simulink model "Palab3_4_2"  (R2025a)
settings: Solver=ode23t  StartTime=0.0  StopTime=10.0  FixedStep=1  MaxStep=1.1  MinStep=0.9  RelTol=1e-3
settings Model: LastModifiedBy=mieszko
settings SolverCC: InitialStep=1

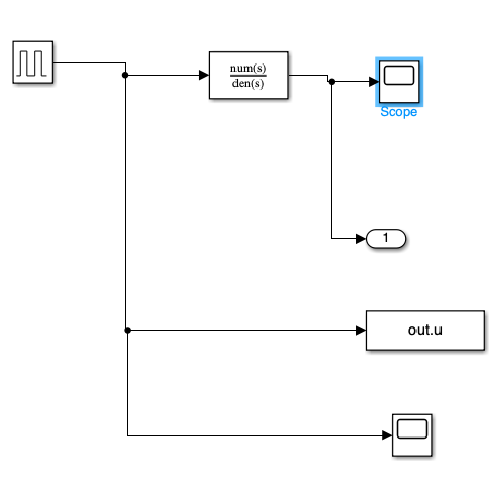
[thumbnail: Simulink's stored preview of the top-level diagram]
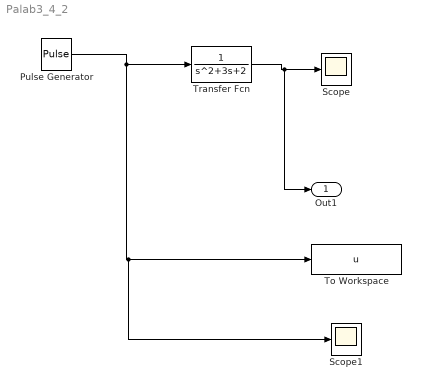
== system Palab3_4_2 ==
  Pulse Generator : DiscretePulseGenerator  PulseType=Time based  PulseWidth=50
  Scope : Scope
      settings: ActiveDisplayYMinimum=-0.63016345231656268  ActiveDisplayYMaximum=1.0718982788419913
  Scope1 : Scope
      settings: ActiveDisplayYMinimum=-0.125  ActiveDisplayYMaximum=1.125
  To Workspace : ToWorkspace  VariableName=u  SampleTime=-1
  Transfer Fcn : TransferFcn  Denominator=[1 3 2]
  Out1 : Outport
  wires:
  Pulse Generator/1 -> Scope1/1, To Workspace/1, Transfer Fcn/1
  Transfer Fcn/1 -> Out1/1, Scope/1
